simulink model "Week1_Q8"  (R2020b)
settings: Solver=VariableStepAuto  StartTime=0.0  StopTime=10.0  RelTol=1e-3
settings Model: Creator=DELL  LastModifiedBy=DELL

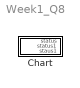
== system Week1_Q8 ==
  Chart : Stateflow chart  TreatAsAtomicUnit=on

== stateflow chart Week1_Q8/Chart ==
  state Ground_Floor
    entry:
    status=1;
    during:
    CurrentFloor=0;
    FloorCheck(CurrentFloor);
    exit:
    status =0;
  state First_Floor
    entry:
    status=1;
    during:
    CurrentFloor=0;
    FloorCheck(CurrentFloor);
    exit:
    status =0;
  state FloorCheck(Floor) [function]
    (default) -> (junction 34)
    (junction 34) -> (junction 33) [order 3] : [FloorSelect<Floor]{
        | send(down);
        | disp('LiftMovingDown');}
    (junction 34) -> (junction 35) [order 1] : [FloorSelect>Floor]{
        | send(up);
        | disp('LiftMovingUp');}
    (junction 33) -> (junction 38)
    (junction 34) -> (junction 37) [order 2] : [FloorSelect==Floor]{
        | disp('CurrentFloor');}
    (junction 35) -> (junction 36)
    (junction 38) -> (junction 37)
    (junction 36) -> (junction 37)
    (junction 37) -> (junction 39)
  state Second_Floor
    entry:
    status=1;
    during:
    CurrentFloor=0;
    FloorCheck(CurrentFloor);
    exit:
    staus =0;
  state Third_Floor
    entry:
    status=1;
    during:
    CurrentFloor=0;
    FloorCheck(CurrentFloor);
    exit:
    status =0;
  state Fourth_Floor
    entry:
    status=1;
    during:
    CurrentFloor=0;
    FloorCheck(CurrentFloor);
    exit:
    status =0;
  state Fifth_Floor
    entry:
    status=1;
    during:
    CurrentFloor=0;
    FloorCheck(CurrentFloor);
    exit:
    status =0;
  (default) -> Ground_Floor
  Ground_Floor -> First_Floor
  First_Floor -> Ground_Floor [order 2]
  First_Floor -> Second_Floor [order 1]
  Second_Floor -> First_Floor [order 2]
  Second_Floor -> Third_Floor [order 1]
  Third_Floor -> Second_Floor [order 2]
  Third_Floor -> Fourth_Floor [order 1]
  Fourth_Floor -> Third_Floor [order 2]
  Fourth_Floor -> Fifth_Floor [order 1]
  Fifth_Floor -> Fourth_Floor
  data: Floor function_input; status output; CurrentFloor local; status1 output; staus1 output; CurrentFloor1 local
